simulink model "tromaseni_model"  (R2023b)
settings: Solver=ode23s  StartTime=0.0  StopTime=Tsim  RelTol=1e-3  EnableMultiTasking=on
values from neighbouring files (symbols this model uses):
  A = [           0       1      0       0      0         0 ... (first row only)    [tmass_ss.m]
  Am = avg_signals1 / 188    [task1.m]
  B = [0 1/m1 0 0 0 0]'    [tmass_ss.m]
  C = [1 0 0 0 0 0 ... (first row only)    [tmass_ss.m]
  D = [0;0;0]    [tmass_ss.m]
  Ts = 0.01    [task1.m]
  Tsim = 2*pi/0.1    (= 62.8318530718)    [task1.m]
undefined symbols (not defined in the file or in its folder): den
libraries: simulink x2
settings Model: Creator=Roadrunner  LastModifiedBy=lvuke
settings SolverCC: AlgebraicLoopSolver=TrustRegion
settings DataIOCC: LimitDataPoints=on  SaveFormat=Array  SignalLoggingSaveFormat=ModelDataLogs  ReturnWorkspaceOutputs=off
settings OptimizationCC: LifeSpan=inf
settings DebuggingCC: UnderspecifiedInitializationDetection=Classic  MergeDetectMultiDrivingBlocksExec=none  SolverPrmCheckMsg=warning  FcnCallInpInsideContextMsg=warning  UnconnectedInputMsg=warning  UnconnectedOutputMsg=warning  UnconnectedLineMsg=warning  AllowSymbolicDim=off  SFUnexpectedBacktrackingDiag=warning  SFNoUnconditionalDefaultTransitionDiag=warning  SFExecutionAtInitializationDiag=none  ArithmeticOperatorsInVariantConditions=warning
settings HardwareCC: ProdBitPerPointer=32  ProdBitPerSizeT=32  ProdBitPerPtrDiffT=32  ProdLargestAtomicFloat=None  ProdIntDivRoundTo=Undefined  ProdEndianess=Unspecified  ProdWordSize=32  ProdHWDeviceType=32-bit Generic
settings ModelReferenceCC: EnableRefExpFcnMdlSchedulingChecks=on  PropagateSignalLabelsOutOfModel=off
settings SFSimCC: SimUseLocalCustomCode=off  CustomCodeUndefinedFunction=UseInterfaceOnly
settings RTWCC: RTWUseLocalCustomCode=off
settings CodeAppCC: StateflowObjectComments=on
settings GRTTargetCC: TargetLangStandard=C89/C90 (ANSI)  CombineOutputUpdateFcns=off  GRTInterface=on
settings ConfigComp: CovMetricSettings=dw  CovSaveCumulativeToWorkspaceVar=on  CovSaveSingleToWorkspaceVar=on  CovExternalEMLEnable=off

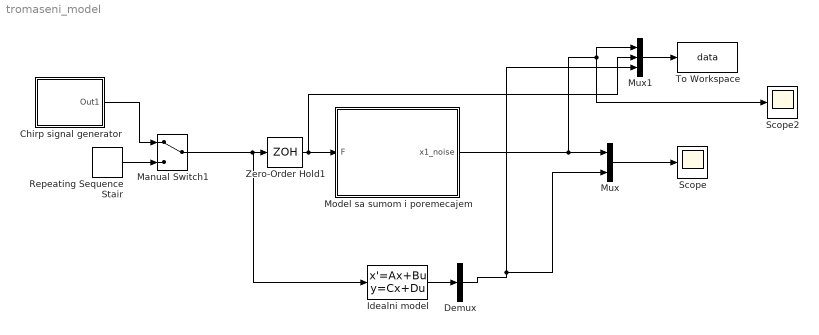
== system tromaseni_model ==
  Chirp signal generator : Subsystem
  Demux : Demux  Outputs=1
  Idealni model : StateSpace  A=A  B=B  C=C  D=D  InitialCondition=0
  Manual Switch1 : ManualSwitch
  Model sa sumom i poremecajem : Subsystem
  Mux : Mux  Inputs=2
  Mux1 : Mux  Inputs=3
  Repeating Sequence Stair : simulink/Sources/Repeating Sequence Stair  OutValues=[3 1 4 2 1].'  tsamp=-1  OutMin=[]  OutMax=[]  OutDataTypeStr=double  OutputDataTypeScalingMode=double  OutDataType=fixdt(0,8)  ConRadixGroup=Best Precision: Vector-wise  OutScaling=2^-12
  Scope : Scope
  Scope2 : Scope
  To Workspace : ToWorkspace  VariableName=data  SaveFormat=Structure With Time  SampleTime=Ts
  Zero-Order Hold1 : ZeroOrderHold  SampleTime=Ts
  wires:
  Model sa sumom i poremecajem/1(x1_noise) -> Scope2/1, Mux1/1, Mux/1
  Mux/1 -> Scope/1
  Mux1/1 -> To Workspace/1
  Idealni model/1 -> Demux/1
  Demux/1 -> Mux1/3, Mux/2
  Manual Switch1/1 -> Idealni model/1, Zero-Order Hold1/1
  Repeating Sequence Stair/1 -> Manual Switch1/2
  Chirp signal generator/1(Out1) -> Manual Switch1/1
  Zero-Order Hold1/1 -> Mux1/2, Model sa sumom i poremecajem/1(F)

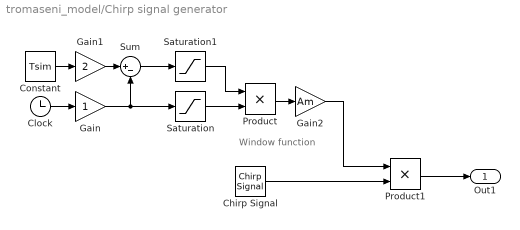
== system tromaseni_model/Chirp signal generator ==
  note: Window function
  Chirp Signal : simulink/Sources/Chirp Signal  f1=0  T=Tsim  f2=10
  Clock : Clock
  Constant : Constant  Value=Tsim
  Gain : Gain
  Gain1 : Gain  Gain=2
  Gain2 : Gain  Gain=Am
  Product : Product
  Product1 : Product
  Saturation : Saturate  UpperLimit=1  LowerLimit=-1
  Saturation1 : Saturate  UpperLimit=1  LowerLimit=-1
  Sum : Sum  Inputs=|+-
  Out1 : Outport
  wires:
  Product1/1 -> Out1/1
  Clock/1 -> Gain/1
  Sum/1 -> Saturation1/1
  Saturation/1 -> Product/2
  Product/1 -> Gain2/1
  Chirp Signal/1 -> Product1/2
  Saturation1/1 -> Product/1
  Constant/1 -> Gain1/1
  Gain/1 -> Saturation/1, Sum/2
  Gain1/1 -> Sum/1
  Gain2/1 -> Product1/1

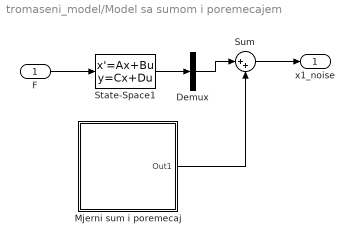
== system tromaseni_model/Model sa sumom i poremecajem ==
  F : Inport
  Demux : Demux  Outputs=1
  Mjerni sum i poremecaj : Subsystem
  State-Space1 : StateSpace  A=A  B=B  C=C  D=D  InitialCondition=0
  Sum : Sum  Inputs=|++
  x1_noise : Outport
  wires:
  F/1 -> State-Space1/1
  Sum/1 -> x1_noise/1
  State-Space1/1 -> Demux/1
  Demux/1 -> Sum/1
  Mjerni sum i poremecaj/1(Out1) -> Sum/2

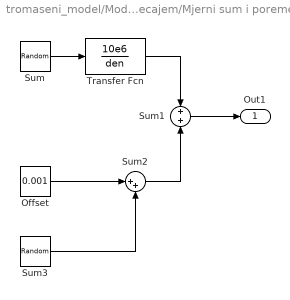
== system tromaseni_model/Model sa sumom i poremecajem/Mjerni sum i poremecaj ==
  Offset : Constant  Value=0.001
  Sum : RandomNumber  Variance=0.00001  SampleTime=0.5
  Sum1 : Sum
  Sum2 : Sum  Inputs=|++
  Sum3 : RandomNumber  Variance=0.00000001  SampleTime=0.001
  Transfer Fcn : TransferFcn  Numerator=[10e6]  Denominator=den
  Out1 : Outport
  wires:
  Sum1/1 -> Out1/1
  Sum/1 -> Transfer Fcn/1
  Offset/1 -> Sum2/1
  Sum2/1 -> Sum1/2
  Transfer Fcn/1 -> Sum1/1
  Sum3/1 -> Sum2/2
